simulink model "StateSpace_Design_Simulation"  (R2022b)
settings: Solver=ode5  StartTime=0.0  StopTime=10  FixedStep=1e-5  RelTol=1e-3
undefined symbols (not defined in the file or in its folder): conv, sf
libraries: simulink x2
settings Model: Creator=gotta  LastModifiedBy=giuliapegoraro
settings SolverCC: ZeroCrossAlgorithm=Adaptive
settings DebuggingCC: IgnoredZcDiagnostic=none
settings SimscapeCC: ExplicitSolverDiagnosticOptions=none

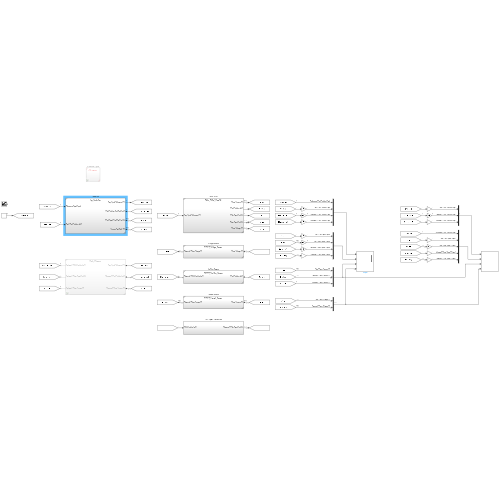
[thumbnail: Simulink's stored preview of the top-level diagram]
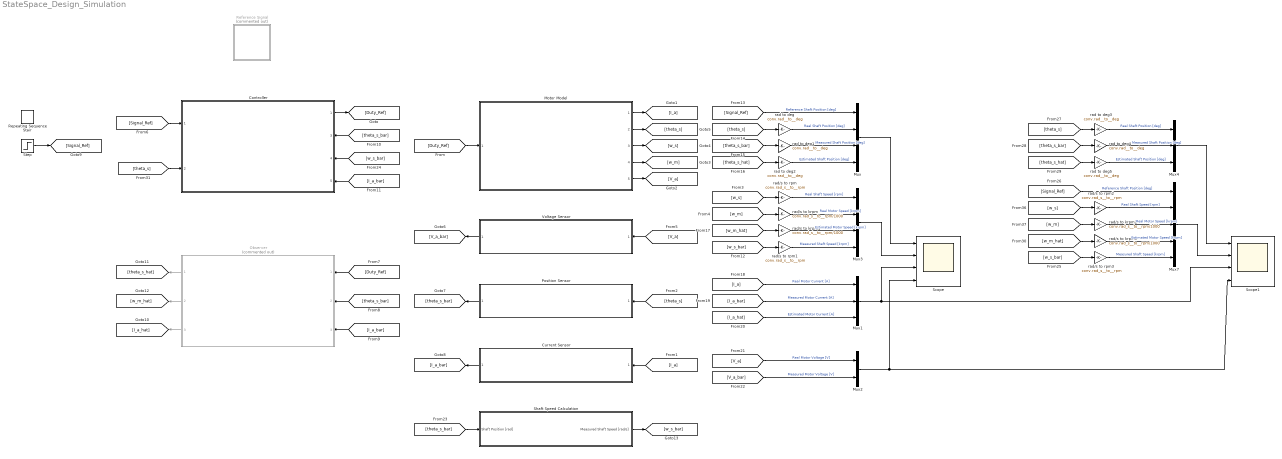
== system StateSpace_Design_Simulation ==
  Controller : Subsystem  ReferencedSubsystem=Lqr_Controller
      settings: PortSchema="{\"entries\":[{\"content\":{\"sides\":[{\"content\":{\"connectorIds\":[\"In1\",\"In2\"]},\"type\":\"ConnectorPlacement.EquallySpacedRectSide\",\"uuid\":\"d5a0e31f-037c-4ee9-822c-85074b9ef060\"},{\"content\":{\"connectorIds\":[\"Out1\",\"In3\",\"In4\",\"In5\"],\"side\":\"RIGHT\"},\"type\":\"ConnectorPlacement.EquallySpacedRectSide\",\"uuid\":\"6f247b27-222f-49ea-af29-336668fb77d8\"},{\"content\":{\"connectorIds\":[],\"side\":\"TOP\"},\"type\":\"ConnectorPlacement.EquallySpacedRectSide\",\"uuid\":\"36e65679-3a56-4a06-8e9a-bcd14510fce9\"}]},\"type\":\"ConnectorPlacement.EquallySpacedConnector\",\"uuid\":\"a3386835-283b-4601-af78-cdf8585604f2\"}],\"packageUris\":[\"http://schema.mathworks.com/mf0/Connector/R2020b\"],\"version\":\"1.0\"}"
  Current Sensor : Subsystem  ReferencedSubsystem=INA219_Current_Sensor
  Motor Model : Subsystem  ReferencedSubsystem=Motor_Model_Simulink
  Mux : Mux
  Mux1 : Mux  Inputs=3
  Mux2 : Mux  Inputs=2
  Mux3 : Mux
  Mux4 : Mux  Inputs=3
  Mux7 : Mux  Inputs=5
  Observer : Subsystem  Commented=on  ReferencedSubsystem=State_Observer
  Position Sensor : Subsystem  ReferencedSubsystem=AS5600_Position_Sensor
  Reference Signal : Subsystem  Commented=on  ReferencedSubsystem=<file name>
  Repeating Sequence Stair : simulink/Sources/Repeating Sequence Stair  OutValues=5*[0 1 2 3 4 5 6 7 8 9]  tsamp=5  OutMin=[]  OutMax=[]  OutDataTypeStr=double  OutputDataTypeScalingMode=double  OutDataType=fixdt(0,8)  ConRadixGroup=Best Precision: Vector-wise  OutScaling=2^-12
  Scope : Scope  NumInputPorts=4
  Scope1 : Scope  NumInputPorts=4
  Shaft Speed Calculation : Subsystem
  Step : Step  Time=0.2  After=10  SampleTime=0
  Voltage Sensor : Subsystem  ReferencedSubsystem=INA219_Voltage_Sensor
  rad to deg{,1..5} (6 alike) : Gain  Gain=conv.rad__to__deg
  rad/s to krpm{,1..3} (4 alike) : Gain  Gain=conv.rad_s__to__rpm/1000
  rad/s to rpm{,1..3} (4 alike) : Gain  Gain=conv.rad_s__to__rpm
  wires:
  rad to deg/1 -> Mux/2  "Real Shaft Position [deg]"
  rad to deg1/1 -> Mux/3  "Measured Shaft Position [deg]"
  rad/s to krpm/1 -> Mux3/2  "Real Motor Speed [krpm]"
  rad/s to rpm/1 -> Mux3/1  "Real Shaft Speed [rpm]"
  rad/s to krpm1/1 -> Mux3/3  "Estimated Motor Speed [krpm]"
  Controller/1 -> [Duty_Ref]
  [Duty_Ref] -> Motor Model/1
  Motor Model/1 -> [I_a]
  Motor Model/2 -> [theta_s]
  Motor Model/5 -> [V_a]
  Motor Model/4 -> [w_m]
  Motor Model/3 -> [w_s]
  [V_a] -> Voltage Sensor/1
  [theta_s] -> Position Sensor/1
  [I_a] -> Current Sensor/1
  Current Sensor/1 -> [I_a_bar]
  Position Sensor/1 -> [theta_s_bar]
  Voltage Sensor/1 -> [V_a_bar]
  [Signal_Ref] -> Controller/1
  [I_a_bar] -> Observer/3
  Observer/1 -> [theta_s_hat]
  Observer/3 -> [I_a_hat]
  Observer/2 -> [w_m_hat]
  [Signal_Ref] -> Mux/1  "Reference Shaft Position [deg]"
  [theta_s] -> rad to deg/1
  [theta_s_bar] -> rad to deg1/1
  [theta_s_hat] -> rad to deg2/1
  rad to deg2/1 -> Mux/4  "Estimated Shaft Position [deg]"
  [w_m_hat] -> rad/s to krpm1/1
  [w_m] -> rad/s to krpm/1
  [w_s] -> rad/s to rpm/1
  [I_a] -> Mux1/1  "Real Motor Current [A]"
  [I_a_bar] -> Mux1/2  "Measured Motor Current [A]"
  [I_a_hat] -> Mux1/3  "Estimated Motor Current [A]"
  [V_a] -> Mux2/1  "Real Motor Voltage [V]"
  [V_a_bar] -> Mux2/2  "Measured Motor Voltage [V]"
  Mux/1 -> Scope/1
  Mux3/1 -> Scope/2
  [Duty_Ref] -> Observer/1
  [theta_s_bar] -> Observer/2
  [theta_s_bar] -> Shaft Speed Calculation/1(Shaft Position [rad])
  [theta_s_bar] -> Controller/3
  [w_s_bar] -> Controller/4
  [I_a_bar] -> Controller/5
  rad/s to rpm1/1 -> Mux3/4  "Measured Shaft Speed [krpm]"
  Shaft Speed Calculation/1(Measured Shaft Speed [rad/s]) -> [w_s_bar]
  [w_s_bar] -> rad/s to rpm1/1
  rad to deg4/1 -> Mux4/2  "Measured Shaft Position [deg]"
  [theta_s_bar] -> rad to deg4/1
  rad/s to krpm2/1 -> Mux7/3  "Real Motor Speed [krpm]"
  rad to deg3/1 -> Mux4/1  "Real Shaft Position [deg]"
  Mux7/1 -> Scope1/2
  [w_s] -> rad/s to rpm2/1
  [theta_s_hat] -> rad to deg5/1
  rad/s to rpm2/1 -> Mux7/2  "Real Shaft Speed [rpm]"
  rad to deg5/1 -> Mux4/3  "Estimated Shaft Position [deg]"
  [w_m] -> rad/s to krpm2/1
  rad/s to rpm3/1 -> Mux7/5  "Measured Shaft Speed [krpm]"
  Mux2/1 -> Scope1/4, Scope/4
  Mux1/1 -> Scope1/3, Scope/3
  [w_m_hat] -> rad/s to krpm3/1
  Mux4/1 -> Scope1/1
  rad/s to krpm3/1 -> Mux7/4  "Estimated Motor Speed [krpm]"
  [theta_s] -> rad to deg3/1
  [w_s_bar] -> rad/s to rpm3/1
  [Signal_Ref] -> Mux7/1  "Reference Shaft Position [deg]"
  Step/1 -> [Signal_Ref]
  [theta_s] -> Controller/2

== system StateSpace_Design_Simulation/Reference Signal ==

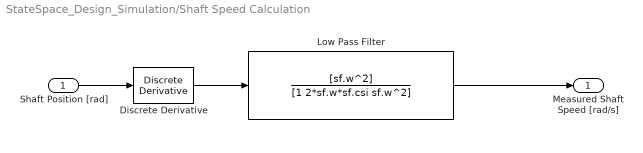
== system StateSpace_Design_Simulation/Shaft Speed Calculation ==
  Shaft Position [rad] : Inport
  Discrete Derivative : simulink/Discrete/Discrete Derivative  gainval=1.0  ICPrevScaledInput=0.0  OutMin=[]  OutMax=[]  OutDataType=fixdt(1, 16)  OutScaling=2^-10  DoSatur=off
  Low Pass Filter : TransferFcn  Numerator=[sf.w^2]  Denominator=[1 2*sf.w*sf.csi sf.w^2]
  Measured Shaft Speed [rad/s] : Outport
  wires:
  Discrete Derivative/1 -> Low Pass Filter/1
  Shaft Position [rad]/1 -> Discrete Derivative/1
  Low Pass Filter/1 -> Measured Shaft Speed [rad/s]/1
